simulink model "Copy_of_Test"  (R2022b)
settings: Solver=FixedStepDiscrete  StartTime=0.0  StopTime=10.0  FixedStep=1e-4  RelTol=1e-3
undefined symbols (not defined in the file): ParamCfg_Avgcnt_u16, ParamCfg_Cosamp_u16, ParamCfg_Cosavg_u16, ParamCfg_Sinamp_u16, ParamCfg_Sinavg_u16, ParamCfg_Stage_u16
libraries: simulink x5
settings Model: DataDictionary=MCU_Input_Sldd.sldd  Creator=ZYH  LastModifiedBy=ZYH
settings OptimizationCC: DefaultParameterBehavior=Inlined  EnhancedBackFolding=on  PassReuseOutputArgsAs=Individual arguments  OptimizeBlockOrder=speed  DifferentSizesBufferReuse=on  OptimizationCustomize=off  EfficientTunableParamExpr=on
settings DebuggingCC: ParameterTunabilityLossMsg=error
settings SFSimCC: MATLABDynamicMemAlloc=off
settings RTWCC: Description=Embedded Coder  SystemTargetFile=ert.tlc  GenCodeOnly=on  TemplateMakefile=ert_default_tmf
settings CodeAppCC: IgnoreCustomStorageClasses=off  MaxIdLength=40  OperatorAnnotations=on  SimulinkDataObjDesc=on  SFDataObjDesc=on  SimulinkBlockComments=off
settings ERTTargetCC: TargetLangStandard=C99 (ISO)  GenerateSampleERTMain=on  InlinedParameterPlacement=NonHierarchical  ERTCustomFileTemplate=example_file_process.tlc

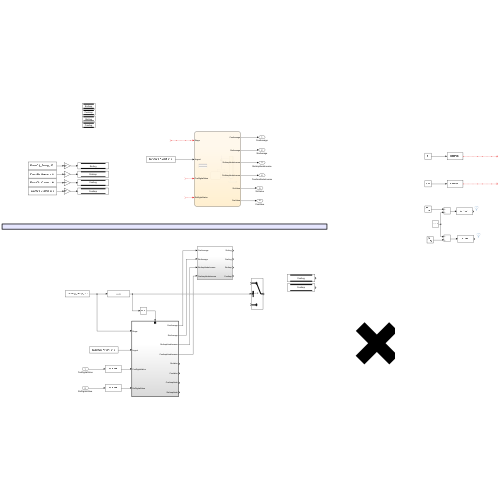
[thumbnail: Simulink's stored preview of the top-level diagram]
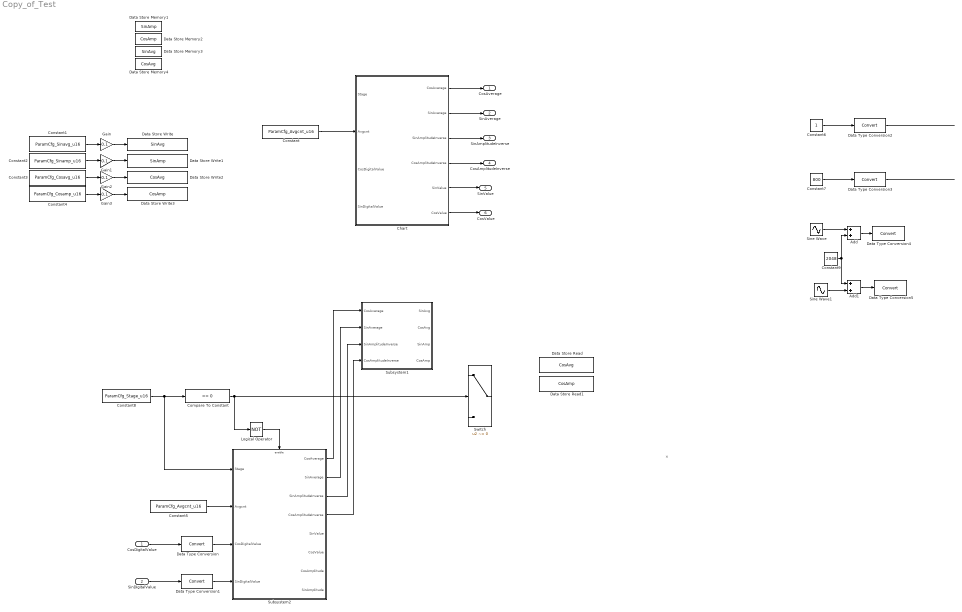
== system Copy_of_Test ==
  note: ✕
  CosDigitalValue : Inport
  SinDigitalValue : Inport  Port=2
  Add : Sum
  Add1 : Sum
  Chart : Stateflow chart  TreatAsAtomicUnit=on
  Compare To Constant : simulink/Logic and Bit Operations/Compare To Constant  relop===  const=0  OutDataTypeStr=boolean
  Constant : Constant  Value=ParamCfg_Avgcnt_u16
  Constant1 : Constant  Value=ParamCfg_Sinavg_u16
  Constant2 : Constant  Value=ParamCfg_Sinamp_u16
  Constant3 : Constant  Value=ParamCfg_Cosavg_u16
  Constant4 : Constant  Value=ParamCfg_Cosamp_u16
  Constant5 : Constant  Value=ParamCfg_Avgcnt_u16
  Constant6 : Constant
  Constant7 : Constant  Value=800
  Constant8 : Constant  Value=ParamCfg_Stage_u16  OutDataTypeStr=uint16
  Constant9 : Constant  Value=2048
  Data Store Memory1 : DataStoreMemory  DataStoreName=SinAmp  WriteAfterWriteMsg=warning  ShowAdditionalParam=off  OutDataTypeStr=single  StateMustResolveToSignalObject=on
  Data Store Memory2 : DataStoreMemory  DataStoreName=CosAmp  WriteAfterWriteMsg=warning  ShowAdditionalParam=off  OutDataTypeStr=single  StateMustResolveToSignalObject=on
  Data Store Memory3 : DataStoreMemory  DataStoreName=SinAvg  WriteAfterWriteMsg=warning  ShowAdditionalParam=off  OutDataTypeStr=single  StateMustResolveToSignalObject=on
  Data Store Memory4 : DataStoreMemory  DataStoreName=CosAvg  WriteAfterWriteMsg=warning  ShowAdditionalParam=off  OutDataTypeStr=single  StateMustResolveToSignalObject=on
  Data Store Read : DataStoreRead  DataStoreName=CosAvg  IndexOptions=Index vector (dialog)  Indices=1  OutputSizes=1
  Data Store Read1 : DataStoreRead  DataStoreName=CosAmp  IndexOptions=Index vector (dialog)  Indices=1  OutputSizes=1
  Data Store Write : DataStoreWrite  DataStoreName=SinAvg  IndexOptions=Index vector (dialog)  Indices=1  OutputSizes=1
  Data Store Write1 : DataStoreWrite  DataStoreName=SinAmp  IndexOptions=Index vector (dialog)  Indices=1  OutputSizes=1
  Data Store Write2 : DataStoreWrite  DataStoreName=CosAvg  IndexOptions=Index vector (dialog)  Indices=1  OutputSizes=1
  Data Store Write3 : DataStoreWrite  DataStoreName=CosAmp  IndexOptions=Index vector (dialog)  Indices=1  OutputSizes=1
  Data Type Conversion{,1..5} (6 alike) : DataTypeConversion  SaturateOnIntegerOverflow=off  RndMeth=Floor
  Gain{,1..3} (4 alike) : Gain  Gain=0.1  ParamDataTypeStr=single  OutDataTypeStr=single
  Logical Operator : Logic  Operator=NOT  AllPortsSameDT=off  OutDataTypeStr=boolean
  Sine Wave : Sin  Amplitude=500  SampleTime=0
  Sine Wave1 : Sin  Amplitude=500  Phase=pi/2  SampleTime=0
  Subsystem1 : Subsystem
  Subsystem2 : Subsystem
  Switch : Switch  Criteria=u2 ~= 0  SaturateOnIntegerOverflow=off  InputSameDT=off
  CosAverage : Outport
  SinAverage : Outport  Port=2
  SinAmplitudeInverse : Outport  Port=3
  CosAmplitudeInverse : Outport  Port=4
  SinValue : Outport  Port=5
  CosValue : Outport  Port=6
  wires:
  ? -> Chart/1(Stage)
  Constant/1 -> Chart/2(Avgcnt)
  CosDigitalValue/1 -> Data Type Conversion/1
  SinDigitalValue/1 -> Data Type Conversion1/1
  ? -> Chart/3(CosDigitalValue)
  ? -> Chart/4(SinDigitalValue)
  Constant1/1 -> Gain/1
  Constant2/1 -> Gain1/1
  Gain/1 -> Data Store Write/1
  Gain1/1 -> Data Store Write1/1
  Constant3/1 -> Gain2/1
  Constant4/1 -> Gain3/1
  Gain2/1 -> Data Store Write2/1
  Gain3/1 -> Data Store Write3/1
  Chart/1(CosAverage) -> CosAverage/1
  Chart/2(SinAverage) -> SinAverage/1
  Chart/3(SinAmplitudeInverse) -> SinAmplitudeInverse/1
  Chart/4(CosAmplitudeInverse) -> CosAmplitudeInverse/1
  Chart/5(SinValue) -> SinValue/1
  Chart/6(CosValue) -> CosValue/1
  Constant8/1 -> Subsystem2/1(Stage), Compare To Constant/1
  Compare To Constant/1 -> Logical Operator/1, Switch/2
  Logical Operator/1 -> Subsystem2/Enable
  Constant5/1 -> Subsystem2/2(Avgcnt)
  Data Type Conversion/1 -> Subsystem2/3(CosDigitalValue)
  Data Type Conversion1/1 -> Subsystem2/4(SinDigitalValue)
  Subsystem2/1(CosAverage) -> Subsystem1/1(CosAverage)
  Subsystem2/2(SinAverage) -> Subsystem1/2(SinAverage)
  Subsystem2/3(SinAmplitudeInverse) -> Subsystem1/3(SinAmplitudeInverse)
  Subsystem2/4(CosAmplitudeInverse) -> Subsystem1/4(CosAmplitudeInverse)
  Data Type Conversion3/1 -> ?
  Add/1 -> Data Type Conversion4/1
  Constant6/1 -> Data Type Conversion2/1
  Sine Wave/1 -> Add/1
  Add1/1 -> Data Type Conversion5/1
  Data Type Conversion2/1 -> ?
  Constant9/1 -> Add/2, Add1/1
  Constant7/1 -> Data Type Conversion3/1
  Sine Wave1/1 -> Add1/2

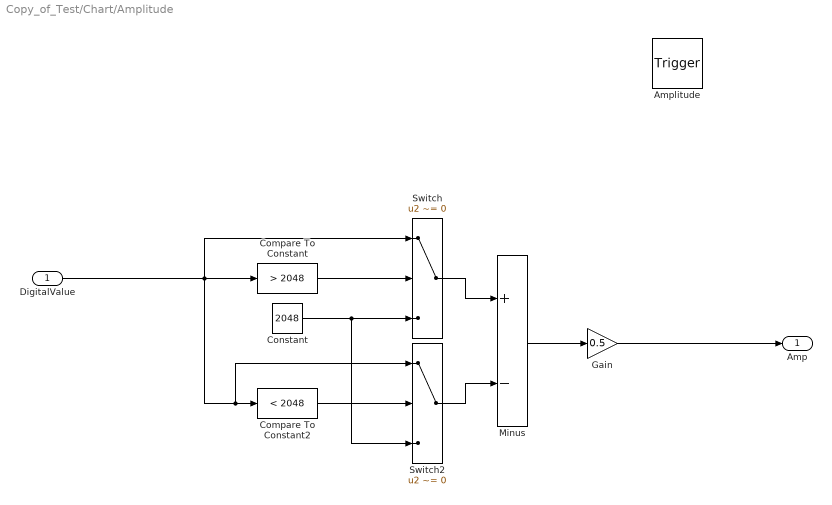
== system Copy_of_Test/Chart/Amplitude ==
  DigitalValue : Inport  OutMin=0  OutMax=65535  OutDataTypeStr=uint16  PortDimensions=1
  Amplitude : TriggerPort  TriggerType=function-call  VariantControl=(inherit)
      settings: CopyFcn=Stateflow.SLINSF.SimulinkMan.removeBlockPreDeleteFcn  PreDeleteFcn=Stateflow.SLINSF.SimulinkMan.unsafePredeleteFcn
  Compare To Constant : simulink/Logic and Bit Operations/Compare To Constant  relop=>  const=2048  OutDataTypeStr=boolean
  Compare To Constant2 : simulink/Logic and Bit Operations/Compare To Constant  relop=<  const=2048  OutDataTypeStr=boolean
  Constant : Constant  Value=2048  OutDataTypeStr=uint16
  Gain : Gain  Gain=0.5  OutDataTypeStr=single
  Minus : Sum  Inputs=+-
  Switch : Switch  Criteria=u2 ~= 0  SaturateOnIntegerOverflow=off  InputSameDT=off
  Switch2 : Switch  Criteria=u2 ~= 0  SaturateOnIntegerOverflow=off  InputSameDT=off
  Amp : Outport  PortDimensions=1
  wires:
  Compare To Constant/1 -> Switch/2
  Gain/1 -> Amp/1
  Compare To Constant2/1 -> Switch2/2
  Switch/1 -> Minus/1
  Switch2/1 -> Minus/2
  Constant/1 -> Switch2/3, Switch/3
  DigitalValue/1 -> Switch2/1, Compare To Constant2/1, Switch/1, Compare To Constant/1
  Minus/1 -> Gain/1

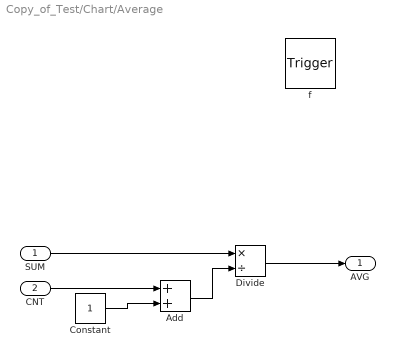
== system Copy_of_Test/Chart/Average ==
  SUM : Inport  OutDataTypeStr=uint32  PortDimensions=1
  CNT : Inport  Port=2  OutDataTypeStr=uint16  PortDimensions=1
  f : TriggerPort  TriggerType=function-call  VariantControl=(inherit)
      settings: CopyFcn=Stateflow.SLINSF.SimulinkMan.removeBlockPreDeleteFcn  PreDeleteFcn=Stateflow.SLINSF.SimulinkMan.unsafePredeleteFcn
  Add : Sum  OutDataTypeStr=uint16
  Constant : Constant  OutDataTypeStr=uint16
  Divide : Product  Inputs=*/  OutDataTypeStr=single
  AVG : Outport  PortDimensions=1
  wires:
  CNT/1 -> Add/1
  Constant/1 -> Add/2
  SUM/1 -> Divide/1
  Add/1 -> Divide/2
  Divide/1 -> AVG/1

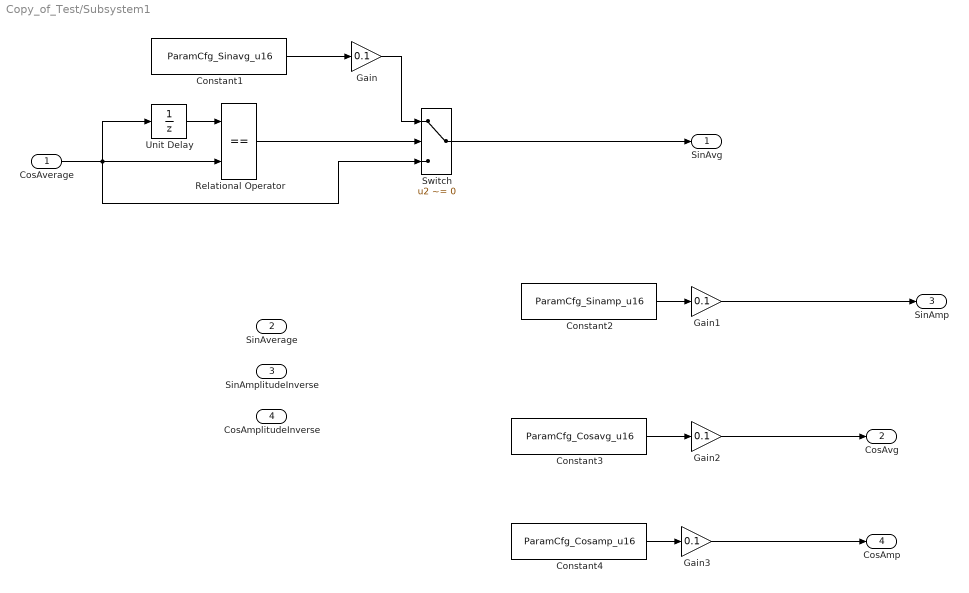
== system Copy_of_Test/Subsystem1 ==
  CosAverage : Inport
  SinAverage : Inport  Port=2
  SinAmplitudeInverse : Inport  Port=3
  CosAmplitudeInverse : Inport  Port=4
  Constant1 : Constant  Value=ParamCfg_Sinavg_u16
  Constant2 : Constant  Value=ParamCfg_Sinamp_u16
  Constant3 : Constant  Value=ParamCfg_Cosavg_u16
  Constant4 : Constant  Value=ParamCfg_Cosamp_u16
  Gain{,1..3} (4 alike) : Gain  Gain=0.1  ParamDataTypeStr=single  OutDataTypeStr=single
  Relational Operator : RelationalOperator  Operator===  OutDataTypeStr=boolean  RndMeth=Simplest  InputSameDT=off
  Switch : Switch  Criteria=u2 ~= 0  SaturateOnIntegerOverflow=off  InputSameDT=off
  Unit Delay : UnitDelay  SampleTime=-1  HasFrameUpgradeWarning=on
  SinAvg : Outport
  CosAvg : Outport  Port=2
  SinAmp : Outport  Port=3
  CosAmp : Outport  Port=4
  wires:
  Constant2/1 -> Gain1/1
  Constant3/1 -> Gain2/1
  Constant1/1 -> Gain/1
  Constant4/1 -> Gain3/1
  Switch/1 -> SinAvg/1
  Gain2/1 -> CosAvg/1
  Gain1/1 -> SinAmp/1
  Gain3/1 -> CosAmp/1
  CosAverage/1 -> Switch/3, Relational Operator/2, Unit Delay/1
  Relational Operator/1 -> Switch/2
  Unit Delay/1 -> Relational Operator/1
  Gain/1 -> Switch/1

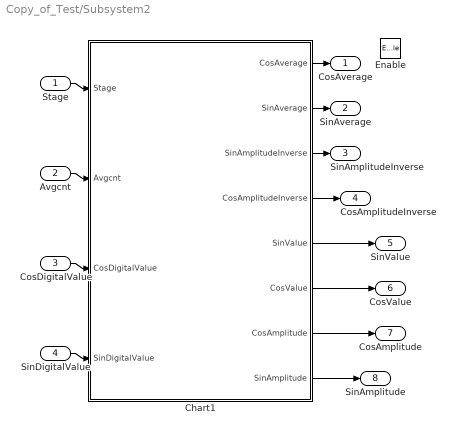
== system Copy_of_Test/Subsystem2 ==
  Stage : Inport
  Avgcnt : Inport  Port=2
  CosDigitalValue : Inport  Port=3
  SinDigitalValue : Inport  Port=4
  Enable : EnablePort
  Chart1 : Stateflow chart  TreatAsAtomicUnit=on
  CosAverage : Outport
  SinAverage : Outport  Port=2
  SinAmplitudeInverse : Outport  Port=3
  CosAmplitudeInverse : Outport  Port=4
  SinValue : Outport  Port=5
  CosValue : Outport  Port=6
  CosAmplitude : Outport  Port=7
  SinAmplitude : Outport  Port=8
  wires:
  Stage/1 -> Chart1/1(Stage)
  Chart1/5(SinValue) -> SinValue/1
  Avgcnt/1 -> Chart1/2(Avgcnt)
  Chart1/2(SinAverage) -> SinAverage/1
  CosDigitalValue/1 -> Chart1/3(CosDigitalValue)
  Chart1/1(CosAverage) -> CosAverage/1
  SinDigitalValue/1 -> Chart1/4(SinDigitalValue)
  Chart1/3(SinAmplitudeInverse) -> SinAmplitudeInverse/1
  Chart1/4(CosAmplitudeInverse) -> CosAmplitudeInverse/1
  Chart1/6(CosValue) -> CosValue/1
  Chart1/7(CosAmplitude) -> CosAmplitude/1
  Chart1/8(SinAmplitude) -> SinAmplitude/1

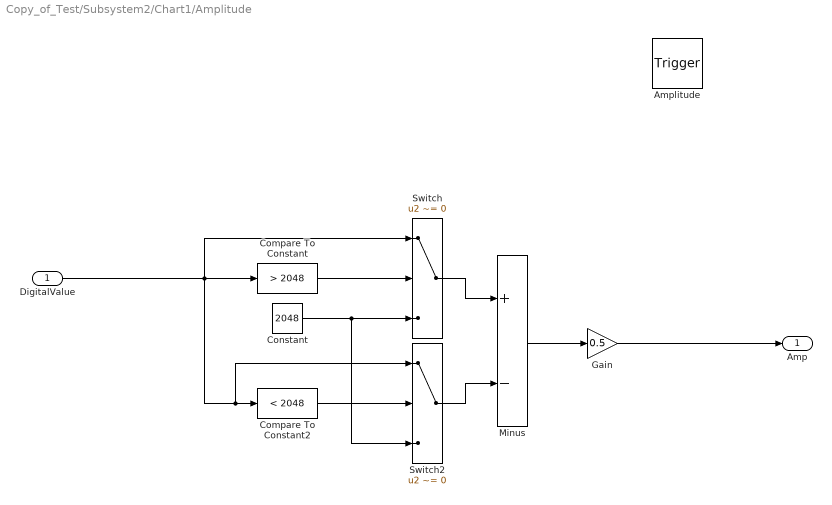
== system Copy_of_Test/Subsystem2/Chart1/Amplitude ==
  DigitalValue : Inport  OutMin=0  OutMax=65535  OutDataTypeStr=uint16  PortDimensions=1
  Amplitude : TriggerPort  TriggerType=function-call  VariantControl=(inherit)
      settings: CopyFcn=Stateflow.SLINSF.SimulinkMan.removeBlockPreDeleteFcn  PreDeleteFcn=Stateflow.SLINSF.SimulinkMan.unsafePredeleteFcn
  Compare To Constant : simulink/Logic and Bit Operations/Compare To Constant  relop=>  const=2048  OutDataTypeStr=boolean
  Compare To Constant2 : simulink/Logic and Bit Operations/Compare To Constant  relop=<  const=2048  OutDataTypeStr=boolean
  Constant : Constant  Value=2048  OutDataTypeStr=uint16
  Gain : Gain  Gain=0.5  OutDataTypeStr=single
  Minus : Sum  Inputs=+-
  Switch : Switch  Criteria=u2 ~= 0  SaturateOnIntegerOverflow=off  InputSameDT=off
  Switch2 : Switch  Criteria=u2 ~= 0  SaturateOnIntegerOverflow=off  InputSameDT=off
  Amp : Outport  PortDimensions=1
  wires:
  Compare To Constant/1 -> Switch/2
  Gain/1 -> Amp/1
  Compare To Constant2/1 -> Switch2/2
  Switch/1 -> Minus/1
  Switch2/1 -> Minus/2
  Constant/1 -> Switch2/3, Switch/3
  DigitalValue/1 -> Switch2/1, Compare To Constant2/1, Switch/1, Compare To Constant/1
  Minus/1 -> Gain/1

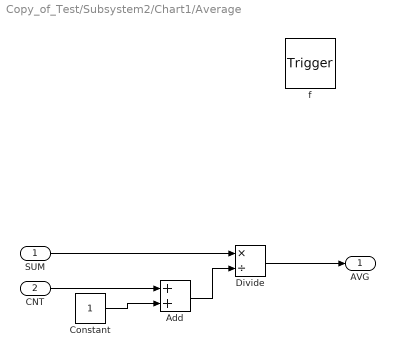
== system Copy_of_Test/Subsystem2/Chart1/Average ==
  SUM : Inport  OutDataTypeStr=uint32  PortDimensions=1
  CNT : Inport  Port=2  OutDataTypeStr=uint16  PortDimensions=1
  f : TriggerPort  TriggerType=function-call  VariantControl=(inherit)
      settings: CopyFcn=Stateflow.SLINSF.SimulinkMan.removeBlockPreDeleteFcn  PreDeleteFcn=Stateflow.SLINSF.SimulinkMan.unsafePredeleteFcn
  Add : Sum  OutDataTypeStr=uint16
  Constant : Constant  OutDataTypeStr=uint16
  Divide : Product  Inputs=*/  OutDataTypeStr=single
  AVG : Outport  PortDimensions=1
  wires:
  CNT/1 -> Add/1
  Constant/1 -> Add/2
  SUM/1 -> Divide/1
  Add/1 -> Divide/2
  Divide/1 -> AVG/1

== stateflow chart Copy_of_Test/Chart ==
  state CalibFinish
    du:
    Cnt = 0;
    SinSum = 0;
    CosSum = 0;
    ToCalibFinish = false;
    ToDown = true;
    end
  state IDLE
  state Amp = Amplitude(DigitalValue) [function]
  state AVG = Average(SUM,CNT) [function]
  state NormlizeSinCos
    du:
    if(Cnt < Avgcnt)
    SinAmplitude = Amplitude(SinDigitalValue);
    CosAmplitude = Amplitude(CosDigitalValue);
    Cnt = Cnt+1;
    SinSum = SinSum + uint32(SinDigitalValue);
    CosSum = CosSum+ uint32(CosDigitalValue);
    else
    SinAverage = Average(SinSum,Cnt);%single(SinSum/(Cnt+1));
    CosAverage = Average(CosSum,Cnt);%single(CosSum/(Cnt+1));
    SinAmplitudeInverse = 1/SinAmplitude;
    CosAmplitudeInverse = 1/CosAmplitude;
    SinAvg = SinAverage*10;
    CosAvg = CosAverage*10;
    SinAmp = SinAmplitude*10;
    CosAmp = CosAmplitude*10;
    end
    ToCalibFinish = true;
    end
  state CompPhaseShift
    SinSum = 1;
    CosSum = 1;
  state Down
    du:
    SinValue = (single(SinDigitalValue)-SinAverage) *SinAmplitudeInverse;
    CosValue = (single(CosDigitalValue)-CosAverage)*CosAmplitudeInverse;
  (default) -> (junction 82)
  (junction 82) -> CalibFinish [order 1] : [Stage == CalibFinish ]
  (junction 82) -> IDLE [order 2]
  IDLE -> (junction 18) : {
      | SinAmplitude = SinAmp;
      | CosAmplitude = CosAmp;
      | SinAverage = SinAvg;
      | CosAverage = CosAvg;
      | SinAmplitudeInverse = 1/SinAmplitude;
      | CosAmplitudeInverse = 1/CosAmplitude;
      | }
  (junction 18) -> (junction 21) [order 1] : [Stage == NormlizeSinCos]
  (junction 18) -> (junction 23) [order 2] : [Stage == CompPhaseShift]
  (junction 21) -> NormlizeSinCos
  (junction 23) -> CompPhaseShift
  NormlizeSinCos -> CalibFinish : [ToCalibFinish ==1]
  CalibFinish -> Down : [ToDown == true]
  data: DigitalValue function_input uint16 size=1; Amp function_output size=1; SUM function_input uint32 size=1; AVG function_output size=1; CNT function_input uint16 size=1; Stage input uint16 size=1; NormlizeSinCos constant uint16 =1; CompPhaseShift constant uint16 =2; CosSum local uint32; Cnt local uint16; SinSum local uint32; Avgcnt input uint16 size=1; CosDigitalValue input uint16 size=1; SinDigitalValue input uint16 size=1; SinAmp data_store_memory; CosAmp data_store_memory; SinAvg data_store_memory; CosAvg data_store_memory; ToCalibFinish local boolean =false; CalibFinish constant uint16 =0; CosAverage output single size=1; SinAverage output single size=1; SinAmplitudeInverse output single size=1; CosAmplitudeInverse output single size=1; CosAmplitude local single; SinAmplitude local single; ToDown local boolean =false; SinValue output; CosValue output

== stateflow chart Copy_of_Test/Subsystem2/Chart1 ==
  state CalibFinish
    du:
    Cnt = 0;
    SinSum = 0;
    CosSum = 0;
    ToCalibFinish = false;
    ToDown = true;
    end
  state IDLE
  state Amp = Amplitude(DigitalValue) [function]
  state AVG = Average(SUM,CNT) [function]
  state NormlizeSinCos
    du:
    if(Cnt < Avgcnt)
    SinAmplitude = Amplitude(SinDigitalValue);
    CosAmplitude = Amplitude(CosDigitalValue);
    Cnt = Cnt+1;
    SinSum = SinSum + uint32(SinDigitalValue);
    CosSum = CosSum+ uint32(CosDigitalValue);
    else
    SinAverage = Average(SinSum,Cnt);%single(SinSum/(Cnt+1));
    CosAverage = Average(CosSum,Cnt);%single(CosSum/(Cnt+1));
    SinAmplitudeInverse = 1/SinAmplitude;
    CosAmplitudeInverse = 1/CosAmplitude;
    SinAvg = SinAverage*10;
    CosAvg = CosAverage*10;
    SinAmp = SinAmplitude*10;
    CosAmp = CosAmplitude*10;
    end
    ToCalibFinish = true;
    end
  state CompPhaseShift
    SinSum = 1;
    CosSum = 1;
  state Down
    du:
    SinValue = (single(SinDigitalValue)-SinAverage) *SinAmplitudeInverse;
    CosValue = (single(CosDigitalValue)-CosAverage)*CosAmplitudeInverse;
  (default) -> (junction 82)
  (junction 82) -> CalibFinish [order 1] : [Stage == CalibFinish ]
  (junction 82) -> IDLE [order 2]
  IDLE -> (junction 18) : {
      | SinAmplitude = SinAmp;
      | CosAmplitude = CosAmp;
      | SinAverage = SinAvg;
      | CosAverage = CosAvg;
      | SinAmplitudeInverse = 1/SinAmplitude;
      | CosAmplitudeInverse = 1/CosAmplitude;
      | }
  (junction 18) -> (junction 21) [order 1] : [Stage == NormlizeSinCos]
  (junction 18) -> (junction 23) [order 2] : [Stage == CompPhaseShift]
  (junction 21) -> NormlizeSinCos
  (junction 23) -> CompPhaseShift
  NormlizeSinCos -> CalibFinish : [ToCalibFinish ==1]
  CalibFinish -> Down : [ToDown == true]
  data: DigitalValue function_input uint16 size=1; Amp function_output size=1; SUM function_input uint32 size=1; AVG function_output size=1; CNT function_input uint16 size=1; Stage input uint16 size=1; NormlizeSinCos constant uint16 =1; CompPhaseShift constant uint16 =2; CosSum local uint32; Cnt local uint16; SinSum local uint32; Avgcnt input uint16 size=1; CosDigitalValue input uint16 size=1; SinDigitalValue input uint16 size=1; SinAmp data_store_memory; CosAmp data_store_memory; SinAvg data_store_memory; CosAvg data_store_memory; ToCalibFinish local boolean =false; CalibFinish constant uint16 =0; CosAverage output single size=1; SinAverage output single size=1; SinAmplitudeInverse output single size=1; CosAmplitudeInverse output single size=1; ToDown local boolean =false; SinValue output; CosValue output; CosAmplitude output single; SinAmplitude output single
